simulink model "foc"  (R2018a)
settings: Solver=VariableStepAuto  StartTime=0.0  StopTime=0.1  RelTol=1e-3
libraries: simulink x1
settings Model: Creator=BOHEMIAN  LastModifiedBy=BOHEMIAN

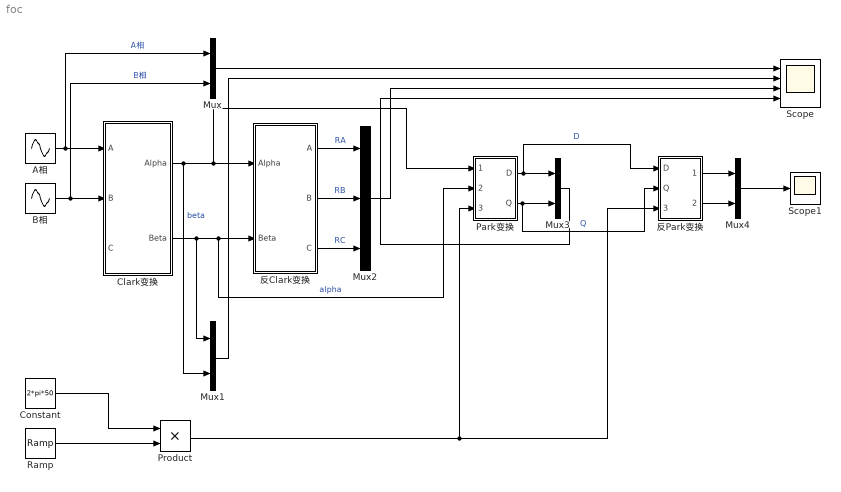
== system foc ==
  A相 : Sin  Frequency=2*pi*50  SampleTime=10e-6
  B相 : Sin  Frequency=2*pi*50  Phase=2*pi/3  SampleTime=10e-6
  Clark变换 : Subsystem
  Constant : Constant  Value=2*pi*50
  Mux{,1,3..4} (4 alike) : Mux  Inputs=2
  Mux2 : Mux  Inputs=3
  Park变换 : Subsystem
  Product : Product
  Ramp : simulink/Sources/Ramp  slope=-1  start=0  InitialOutput=0
  Scope : Scope  NumInputPorts=4
  Scope1 : Scope
  反Clark变换 : Subsystem
  反Park变换 : Subsystem
  wires:
  A相/1 -> Mux/1, Clark变换/1(A)  "A相"
  B相/1 -> Mux/2, Clark变换/2(B)  "B相"
  Clark变换/1(Alpha) -> Park变换/1(Alpha), 反Clark变换/1(Alpha), Mux1/2  "beta"
  Clark变换/2(Beta) -> Mux1/1, Park变换/2(Beta), 反Clark变换/2(Beta)  "alpha"
  Mux/1 -> Scope/1
  Mux1/1 -> Scope/2
  反Clark变换/1(A) -> Mux2/1  "RA"
  反Clark变换/2(B) -> Mux2/2  "RB"
  反Clark变换/3(C) -> Mux2/3  "RC"
  Mux2/1 -> Scope/3
  Park变换/1(D) -> 反Park变换/1(D), Mux3/1  "D"
  Park变换/2(Q) -> 反Park变换/2(Q), Mux3/2  "Q"
  Mux3/1 -> Scope/4
  反Park变换/1(Alpha) -> Mux4/1
  反Park变换/2(Beta) -> Mux4/2
  Mux4/1 -> Scope1/1
  Ramp/1 -> Product/2
  Constant/1 -> Product/1
  Product/1 -> 反Park变换/3(The), Park变换/3(theta)

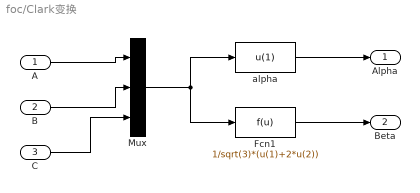
== system foc/Clark变换 ==
  A : Inport
  B : Inport  Port=2
  C : Inport  Port=3
  Fcn1 : Fcn  Expr=1/sqrt(3)*(u(1)+2*u(2))
  Mux : Mux  Inputs=3
  alpha : Fcn  Expr=u(1)
  Alpha : Outport
  Beta : Outport  Port=2
  wires:
  Mux/1 -> Fcn1/1, alpha/1
  A/1 -> Mux/1
  alpha/1 -> Alpha/1
  B/1 -> Mux/2
  Fcn1/1 -> Beta/1
  C/1 -> Mux/3

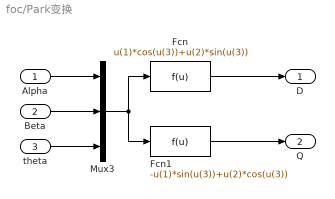
== system foc/Park变换 ==
  Alpha : Inport
  Beta : Inport  Port=2
  theta : Inport  Port=3
  Fcn : Fcn  Expr=u(1)*cos(u(3))+u(2)*sin(u(3))
  Fcn1 : Fcn  Expr=-u(1)*sin(u(3))+u(2)*cos(u(3))
  Mux3 : Mux  Inputs=3
  D : Outport
  Q : Outport  Port=2
  wires:
  Fcn/1 -> D/1
  Mux3/1 -> Fcn1/1, Fcn/1
  Fcn1/1 -> Q/1
  theta/1 -> Mux3/3
  Beta/1 -> Mux3/2
  Alpha/1 -> Mux3/1

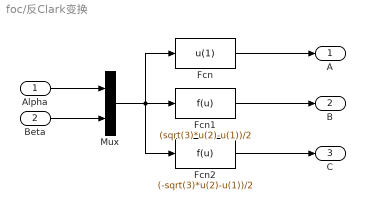
== system foc/反Clark变换 ==
  Alpha : Inport
  Beta : Inport  Port=2
  Fcn : Fcn  Expr=u(1)
  Fcn1 : Fcn  Expr=(sqrt(3)*u(2)-u(1))/2
  Fcn2 : Fcn  Expr=(-sqrt(3)*u(2)-u(1))/2
  Mux : Mux  Inputs=2
  A : Outport
  B : Outport  Port=2
  C : Outport  Port=3
  wires:
  Fcn/1 -> A/1
  Mux/1 -> Fcn2/1, Fcn1/1, Fcn/1
  Beta/1 -> Mux/2
  Alpha/1 -> Mux/1
  Fcn1/1 -> B/1
  Fcn2/1 -> C/1

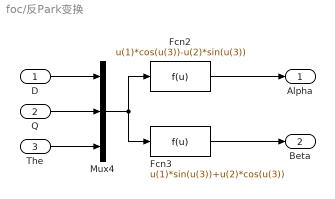
== system foc/反Park变换 ==
  D : Inport
  Q : Inport  Port=2
  The : Inport  Port=3
  Fcn2 : Fcn  Expr=u(1)*cos(u(3))-u(2)*sin(u(3))
  Fcn3 : Fcn  Expr=u(1)*sin(u(3))+u(2)*cos(u(3))
  Mux4 : Mux  Inputs=3
  Alpha : Outport
  Beta : Outport  Port=2
  wires:
  D/1 -> Mux4/1
  Mux4/1 -> Fcn3/1, Fcn2/1
  Q/1 -> Mux4/2
  Fcn3/1 -> Beta/1
  Fcn2/1 -> Alpha/1
  The/1 -> Mux4/3
